simulink model "Ejercicio_9"  (R2013a)
settings: Solver=ode45  StartTime=0.0  StopTime=10  RelTol=1e-3
libraries: simulink x1
settings Model: Creator=Miguel  LastModifiedBy=Miguel

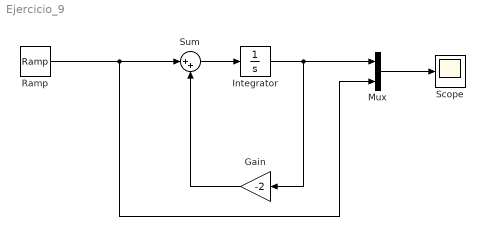
== system Ejercicio_9 ==
  Gain : Gain  Gain=-2
  Integrator : Integrator
  Mux : Mux  Inputs=2
  Ramp : simulink/Sources/Ramp  slope=1  start=0  X0=0
  Scope : Scope
      settings: ShowLegends=on
  Sum : Sum  Inputs=|++
  wires:
  Mux/1 -> Scope/1
  Sum/1 -> Integrator/1
  Integrator/1 -> Gain/1, Mux/1
  Ramp/1 -> Mux/2, Sum/1
  Gain/1 -> Sum/2
